simulink model "Model"  (R2017b)
settings: Solver=VariableStepAuto  StartTime=0.0  StopTime=40000  RelTol=1e-3
undefined symbols (not defined in the file or in its folder): f, J, Ke, Kt, L, Mb, P, r, R
settings Model: Creator=asger  LastModifiedBy=asger

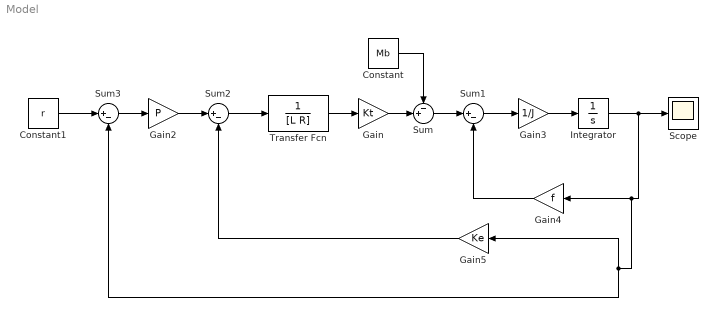
== system Model ==
  Constant : Constant  Value=Mb
  Constant1 : Constant  Value=r
  Gain : Gain  Gain=Kt
  Gain2 : Gain  Gain=P
  Gain3 : Gain  Gain=1/J
  Gain4 : Gain  Gain=f
  Gain5 : Gain  Gain=Ke
  Integrator : Integrator
  Scope : Scope
  Sum : Sum  Inputs=-+|
  Sum1 : Sum  Inputs=|+-
  Sum2 : Sum  Inputs=|+-
  Sum3 : Sum  Inputs=|+-
  Transfer Fcn : TransferFcn  Denominator=[L R]  ContinuousStateAttributes='uh'
  wires:
  Gain/1 -> Sum/2
  Sum/1 -> Sum1/1
  Sum3/1 -> Gain2/1
  Gain2/1 -> Sum2/1
  Sum1/1 -> Gain3/1
  Gain3/1 -> Integrator/1
  Integrator/1 -> Sum3/2, Gain5/1, Gain4/1, Scope/1
  Gain4/1 -> Sum1/2
  Gain5/1 -> Sum2/2
  Constant/1 -> Sum/1
  Constant1/1 -> Sum3/1
  Transfer Fcn/1 -> Gain/1
  Sum2/1 -> Transfer Fcn/1
